simulink model "Regressao6_Comp"  (R2012b)
settings: Solver=FixedStepDiscrete  SolverMode=SingleTasking  StartTime=0.0  StopTime=buffer*limSim  FixedStep=ts  RelTol=1e-3
undefined symbols (not defined in the file): buffer, limSim, magnitude, ts
libraries: xbsIndex_r4 x52, dspstat3 x1, simulink x1, roblocks x1
settings Model: Creator=snata  LastModifiedBy=snata

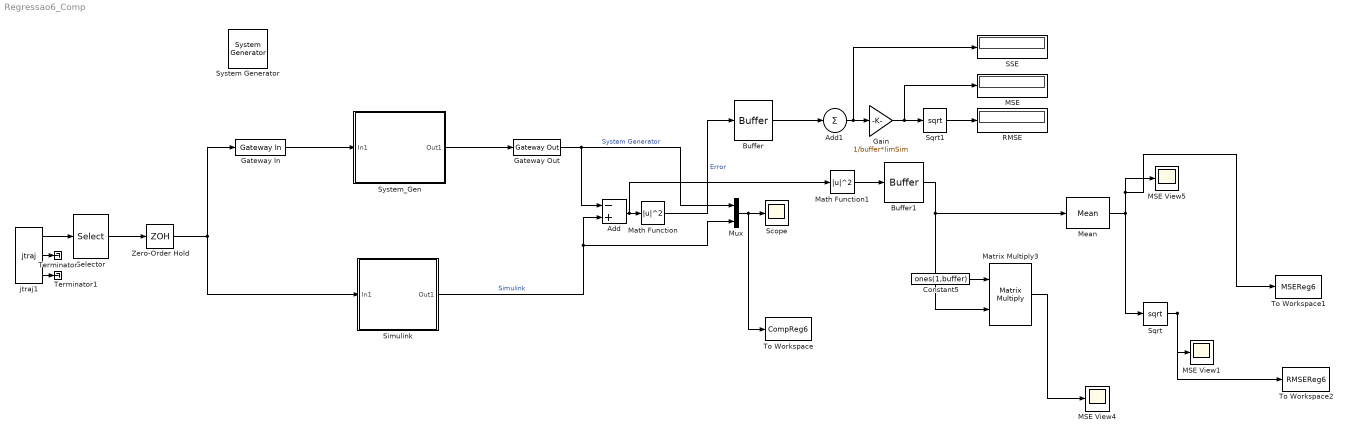
== system Regressao6_Comp ==
  " System Generator" : xbsIndex_r4/ System Generator  Tag=genX  xilinxfamily=virtex6  part=xc6vlx240t  speed=-1  package=ff1156  synthesis_tool=XST  clock_wrapper=Clock Enables  directory=./netlist  proj_type=Project Navigator  Synth_file=XST Defaults  Impl_file=ISE Defaults  testbench=off  simulink_period=ts  sysclk_period=10  dcm_input_clock_period=10  incr_netlist=off  trim_vbits=Everywhere in SubSystem  dbl_ovrd=According to Block Masks  core_generation=According to Block Masks  run_coregen=off  deprecated_control=off  eval_field=0  block_type=sysgen
  Add : Sum  Inputs=-+
  Add1 : Sum  Inputs=1
  Buffer : Buffer  N=buffer*limSim  TreatMby1Signals=One channel
  Buffer1 : Buffer  N=buffer  TreatMby1Signals=One channel
  Constant5 : Constant  Value=ones(1,buffer)  VectorParams1D=off
  Gain : Gain  Gain=1/buffer*limSim
  Gateway In : xbsIndex_r4/Gateway In  gui_display_data_type=Floating-point  arith_type=Floating-point  n_bits=16  bin_pt=14  preci_type=Single  exp_width=8  frac_width=24  quantization="Round  (unbiased: +/- Inf)"  overflow=Saturate  period=ts  dbl_ovrd=off  timing_constraint=None  locs_specified=off  LOCs={}  UseAsADC=off  ADCChannel='1'  inherit_from_input=off  hdl_port=on  block_type=gatewayin
  Gateway Out : xbsIndex_r4/Gateway Out  inherit_from_input=off  hdl_port=on  timing_constraint=None  locs_specified=off  LOCs={}  UseAsDAC=off  DACChannel='1'  block_type=gatewayout
  MSE : Display
  MSE View1 : Scope
      settings: TimeRange=1600  YMin=0.3388218390804599  YMax=0.5988218390804599  SaveName=ScopeData4  MaxDataPoints=5000000
  MSE View4 : Scope
      settings: TimeRange=1600  YMin=0.3388218390804599  YMax=0.5988218390804599  SaveName=ScopeData5  MaxDataPoints=5000000
  MSE View5 : Scope
      settings: ShowLegends=on  TimeRange=4000  YMin=0.3388218390804599  YMax=0.5988218390804599  SaveName=ScopeData6  MaxDataPoints=5000000
  Math Function1 : Math  Operator=magnitude^2  SaturateOnIntegerOverflow=on
  Math Function : Math  Operator=magnitude^2  SaturateOnIntegerOverflow=on
  Matrix Multiply3 : Product  Multiplication=Matrix(*)
  Mean : dspstat3/Mean  run=off  reset_popup=None  InputProcessing=Columns as channels (frame based)  directionMode=Each column  dimension=1  treatSBRowAsCol=on  roiEnable=off  roiType=Rectangles  roiPortion=Entire ROI  roiOutput=Individual statistics for each ROI  roiFlag=off  outputDataTypeStr=Inherit: Same as accumulator  outputLastDataTypeStr=Inherit: Same as accumulator  outputMin=[]  outputMax=[]  roundingMode=Floor  overflowMode=off
  Mux : Mux  Inputs=2
  RMSE : Display
  SSE : Display
  Scope : Scope
      settings: ShowLegends=on  TimeRange=40  YMin=0  YMax=200  MaxDataPoints=50000
  Selector : Selector  InputPortWidth=3  IndexOptions=Index vector (dialog)  Indices=[1]  OutputSizes=1
  Simulink : Subsystem
  Sqrt : Sqrt  SaturateOnIntegerOverflow=on
  Sqrt1 : Sqrt  SaturateOnIntegerOverflow=on
  System_Gen : Subsystem
  Terminator : Terminator
  Terminator1 : Terminator
  To Workspace : ToWorkspace  VariableName=CompReg6  SampleTime=-1
  To Workspace1 : ToWorkspace  VariableName=MSEReg6  SampleTime=-1
  To Workspace2 : ToWorkspace  VariableName=RMSEReg6  SampleTime=-1
  Zero-Order Hold : ZeroOrderHold  SampleTime=ts
  jtraj1 : roblocks/Trajectory/jtraj  q0=[0 -pi/2 pi]  qf=[pi/2 pi/4 pi/2]  tmax=buffer*limSim  ts=ts
  wires:
  Selector/1 -> Zero-Order Hold/1
  jtraj1/1 -> Selector/1
  Gateway In/1 -> System_Gen/1(In1)
  System_Gen/1(Out1) -> Gateway Out/1
  Gateway Out/1 -> Add/1, Mux/1  "System Generator"
  Simulink/1(Out1) -> Mux/2, Add/2  "Simulink"
  Zero-Order Hold/1 -> Gateway In/1, Simulink/1(In1)
  Math Function/1 -> Buffer/1  "Error"
  Gain/1 -> MSE/1, Sqrt1/1
  Buffer/1 -> Add1/1
  Add1/1 -> SSE/1, Gain/1
  Sqrt1/1 -> RMSE/1
  jtraj1/2 -> Terminator/1
  jtraj1/3 -> Terminator1/1
  Mux/1 -> To Workspace/1, Scope/1
  Add/1 -> Math Function1/1, Math Function/1
  Math Function1/1 -> Buffer1/1
  Buffer1/1 -> Mean/1, Matrix Multiply3/2
  Matrix Multiply3/1 -> MSE View4/1
  Constant5/1 -> Matrix Multiply3/1
  Mean/1 -> To Workspace1/1, MSE View5/1, Sqrt/1
  Sqrt/1 -> To Workspace2/1, MSE View1/1

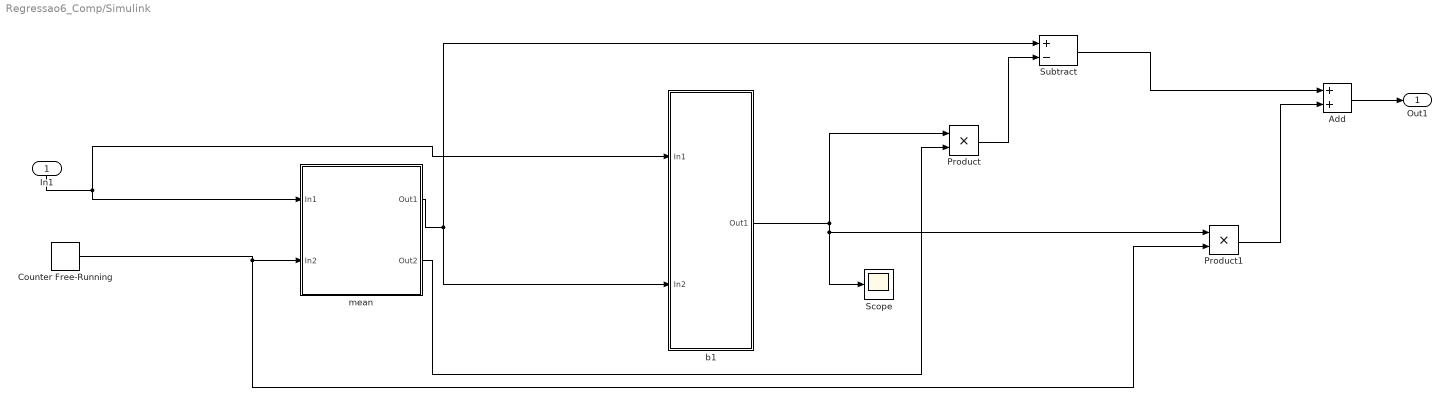
== system Regressao6_Comp/Simulink ==
  In1 : Inport
  Add : Sum
  Counter Free-Running : simulink/Sources/Counter Free-Running  NumBits=32  tsamp=ts
  Product : Product  RndMeth=Zero
  Product1 : Product  RndMeth=Zero
  Scope : Scope
      settings: ShowLegends=on  TimeRange=40  YMin=2.88  YMax=2.945  SaveName=ScopeData3  MaxDataPoints=50000
  Subtract : Sum  Inputs=+-
  b1 : Subsystem
  "mean " : Subsystem
  Out1 : Outport
  wires:
  Subtract/1 -> Add/1
  In1/1 -> "mean "/1(In1), b1/1(In1)
  Add/1 -> Out1/1
  "mean "/1(Out1) -> Subtract/1, b1/2(In2)
  b1/1(Out1) -> Scope/1, Product1/1, Product/1
  Counter Free-Running/1 -> "mean "/2(In2), Product1/2
  "mean "/2(Out2) -> Product/2
  Product/1 -> Subtract/2
  Product1/1 -> Add/2

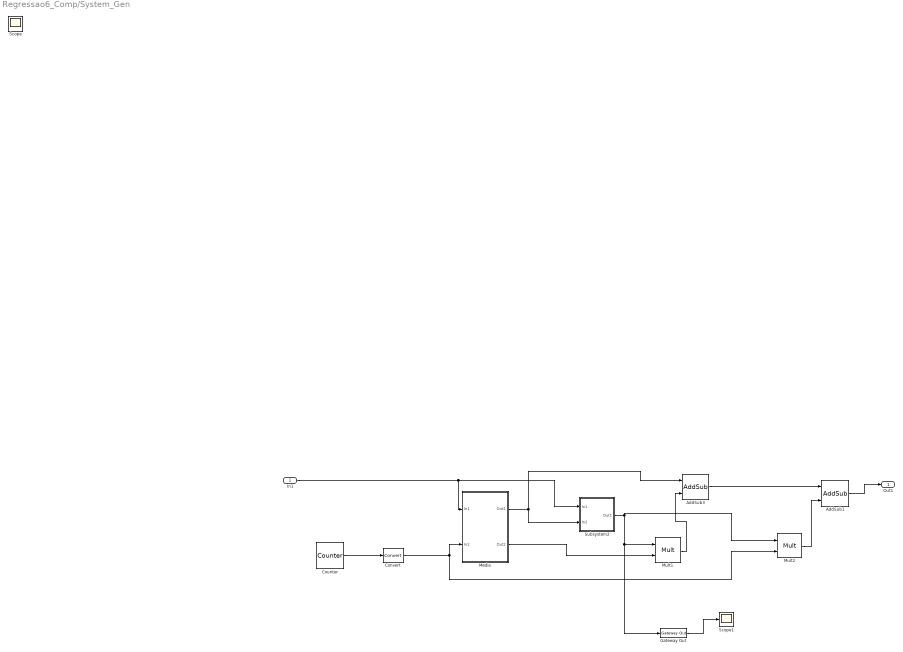
== system Regressao6_Comp/System_Gen ==
  In1 : Inport
  AddSub1 : xbsIndex_r4/AddSub  mode=Addition  use_carryin=off  use_carryout=off  en=off  latency=0  precision=Full  arith_type=Unsigned  n_bits=16  bin_pt=14  quantization=Truncate  overflow=Wrap  dbl_ovrd=off  use_behavioral_HDL=off  hw_selection=Fabric  pipelined=off  block_type=addsub
  AddSub3 : xbsIndex_r4/AddSub  mode=Subtraction  use_carryin=off  use_carryout=off  en=off  latency=0  precision=Full  arith_type=Unsigned  n_bits=16  bin_pt=14  quantization=Truncate  overflow=Wrap  dbl_ovrd=off  use_behavioral_HDL=off  hw_selection=Fabric  pipelined=off  block_type=addsub
  Convert : xbsIndex_r4/Convert  gui_display_data_type=Floating-point  arith_type=Floating-point  n_bits=16  bin_pt=14  float_type=Single  exp_bits=8  fraction_bits=24  quantization=Truncate  overflow=Wrap  en=off  latency=0  dbl_ovrd=off  pipeline=off  block_type=convert
  Counter : xbsIndex_r4/Counter  cnt_type=Free Running  cnt_to=Inf  operation=Up  start_count=0  cnt_by_val=1  arith_type="Signed  (2's comp)"  n_bits=32  bin_pt=0  load_pin=off  rst=off  en=off  explicit_period=on  period=ts  dbl_ovrd=off  use_behavioral_HDL=off  implementation=Fabric  block_type=counter
  Gateway Out : xbsIndex_r4/Gateway Out  inherit_from_input=off  hdl_port=on  timing_constraint=None  locs_specified=off  LOCs={}  UseAsDAC=off  DACChannel='1'  block_type=gatewayout
  "Media " : Subsystem
  Mult1 : xbsIndex_r4/Mult  precision=Full  arith_type="Signed  (2's comp)"  n_bits=16  bin_pt=14  quantization=Truncate  overflow=Wrap  en=off  latency=0  dbl_ovrd=off  use_behavioral_HDL=off  opt=Speed  use_embedded=on  optimum_pipeline=off  pipeline=on  use_rpm=on  placement_style=Triangular  block_type=mult
  Mult2 : xbsIndex_r4/Mult  precision=Full  arith_type="Signed  (2's comp)"  n_bits=16  bin_pt=14  quantization=Truncate  overflow=Wrap  en=off  latency=0  dbl_ovrd=off  use_behavioral_HDL=off  opt=Speed  use_embedded=on  optimum_pipeline=off  pipeline=on  use_rpm=on  placement_style=Triangular  block_type=mult
  Scope : Scope
      settings: ShowLegends=on  TimeRange=40  YMin=0  YMax=200  MaxDataPoints=50000
  Scope1 : Scope
      settings: ShowLegends=on  TimeRange=40  YMin=0  YMax=200  SaveName=ScopeData2  MaxDataPoints=50000
  Subsystem2 : Subsystem
  Out1 : Outport
  wires:
  AddSub1/1 -> Out1/1
  In1/1 -> Subsystem2/1(In1), "Media "/1(In1)
  "Media "/1(Out1) -> Subsystem2/2(In2), AddSub3/1
  Mult1/1 -> AddSub3/2
  AddSub3/1 -> AddSub1/1
  Mult2/1 -> AddSub1/2
  Subsystem2/1(Out1) -> Mult2/1, Gateway Out/1, Mult1/1
  "Media "/2(Out2) -> Mult1/2
  Counter/1 -> Convert/1
  Convert/1 -> "Media "/2(In2), Mult2/2
  Gateway Out/1 -> Scope1/1

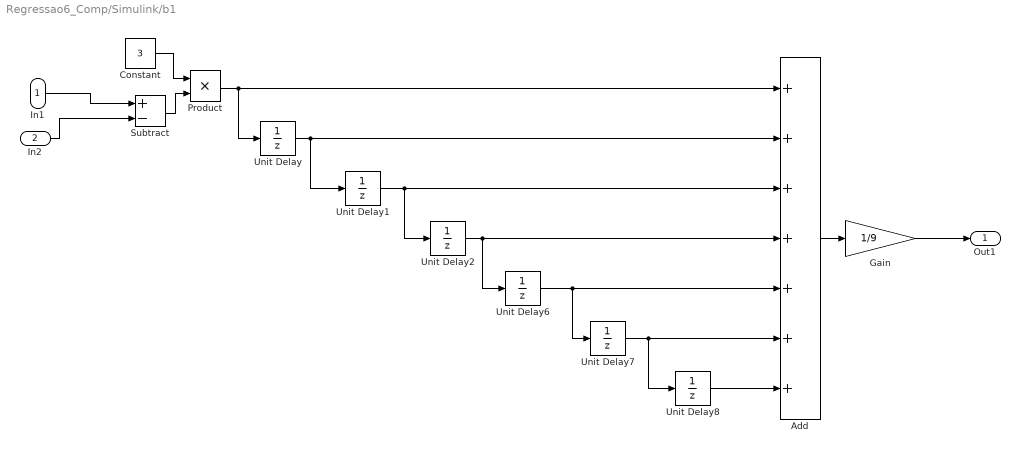
== system Regressao6_Comp/Simulink/b1 ==
  In1 : Inport
  In2 : Inport  Port=2
  Add : Sum  Inputs=+++++++
  Constant : Constant  Value=3
  Gain : Gain  Gain=1/9
  Product : Product
  Subtract : Sum  Inputs=+-
  Unit Delay{,1..2,6..8} (6 alike) : UnitDelay  SampleTime=-1
  Out1 : Outport
  wires:
  In1/1 -> Subtract/1
  Gain/1 -> Out1/1
  In2/1 -> Subtract/2
  Subtract/1 -> Product/2
  Add/1 -> Gain/1
  Constant/1 -> Product/1
  Unit Delay8/1 -> Add/7
  Unit Delay7/1 -> Unit Delay8/1, Add/6
  Unit Delay6/1 -> Unit Delay7/1, Add/5
  Unit Delay2/1 -> Unit Delay6/1, Add/4
  Unit Delay1/1 -> Unit Delay2/1, Add/3
  Unit Delay/1 -> Unit Delay1/1, Add/2
  Product/1 -> Unit Delay/1, Add/1

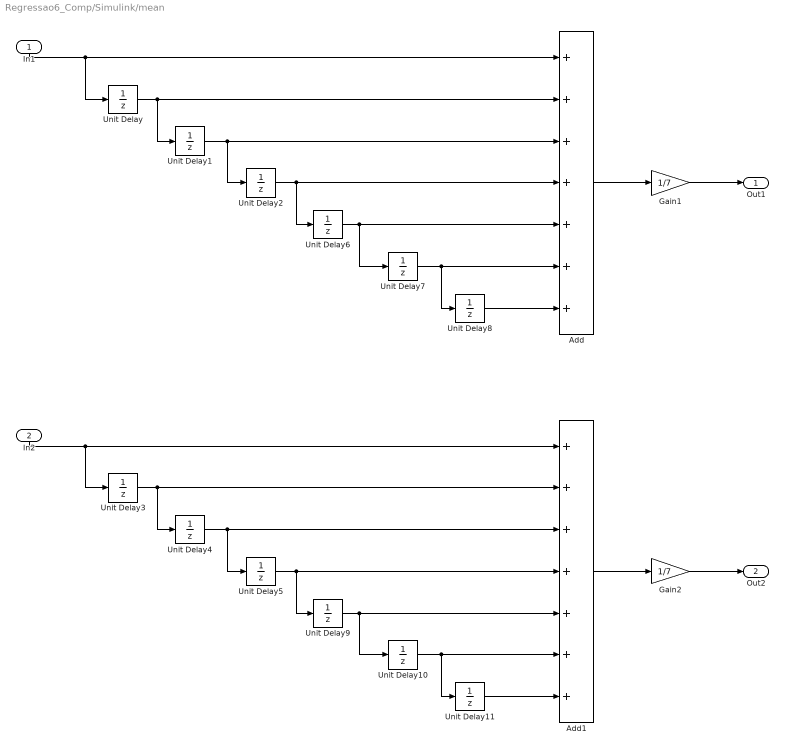
== system Regressao6_Comp/Simulink/mean  ==
  In1 : Inport
  In2 : Inport  Port=2
  Add : Sum  Inputs=+++++++
  Add1 : Sum  Inputs=+++++++
  Gain1 : Gain  Gain=1/7
  Gain2 : Gain  Gain=1/7
  Unit Delay{,1..11} (12 alike) : UnitDelay  SampleTime=-1
  Out1 : Outport
  Out2 : Outport  Port=2
  wires:
  Gain1/1 -> Out1/1
  Add/1 -> Gain1/1
  Unit Delay8/1 -> Add/7
  Unit Delay7/1 -> Unit Delay8/1, Add/6
  Unit Delay6/1 -> Unit Delay7/1, Add/5
  Unit Delay2/1 -> Unit Delay6/1, Add/4
  Unit Delay1/1 -> Unit Delay2/1, Add/3
  Unit Delay/1 -> Unit Delay1/1, Add/2
  In1/1 -> Unit Delay/1, Add/1
  Gain2/1 -> Out2/1
  Add1/1 -> Gain2/1
  Unit Delay11/1 -> Add1/7
  Unit Delay10/1 -> Add1/6, Unit Delay11/1
  Unit Delay9/1 -> Add1/5, Unit Delay10/1
  Unit Delay5/1 -> Add1/4, Unit Delay9/1
  Unit Delay4/1 -> Add1/3, Unit Delay5/1
  Unit Delay3/1 -> Add1/2, Unit Delay4/1
  In2/1 -> Add1/1, Unit Delay3/1

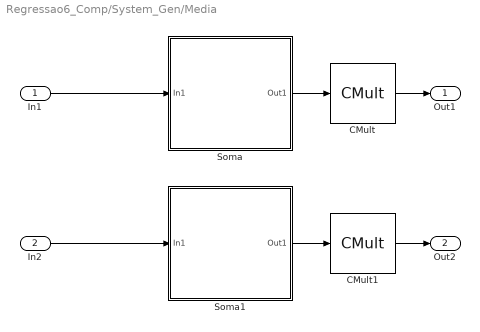
== system Regressao6_Comp/System_Gen/Media  ==
  In1 : Inport
  In2 : Inport  Port=2
  CMult : xbsIndex_r4/CMult  const=1/7  gui_display_data_type=Floating-point  const_n_bits=16  const_bin_pt=14  float_type=Single  exp_bits=8  fraction_bits=24  en=off  latency=0  precision=Full  arith_type="Signed  (2's comp)"  n_bits=16  bin_pt=14  quantization=Truncate  overflow=Wrap  dbl_ovrd=off  use_behavioral_HDL=off  mem_type=Distributed RAM  pipeline=off  block_type=cmult
  CMult1 : xbsIndex_r4/CMult  const=1/7  gui_display_data_type=Floating-point  const_n_bits=16  const_bin_pt=14  float_type=Single  exp_bits=8  fraction_bits=24  en=off  latency=0  precision=Full  arith_type="Signed  (2's comp)"  n_bits=16  bin_pt=14  quantization=Truncate  overflow=Wrap  dbl_ovrd=off  use_behavioral_HDL=off  mem_type=Distributed RAM  pipeline=off  block_type=cmult
  Soma : Subsystem
  Soma1 : Subsystem
  Out1 : Outport
  Out2 : Outport  Port=2
  wires:
  In1/1 -> Soma/1(In1)
  Soma/1(Out1) -> CMult/1
  CMult/1 -> Out1/1
  In2/1 -> Soma1/1(In1)
  Soma1/1(Out1) -> CMult1/1
  CMult1/1 -> Out2/1

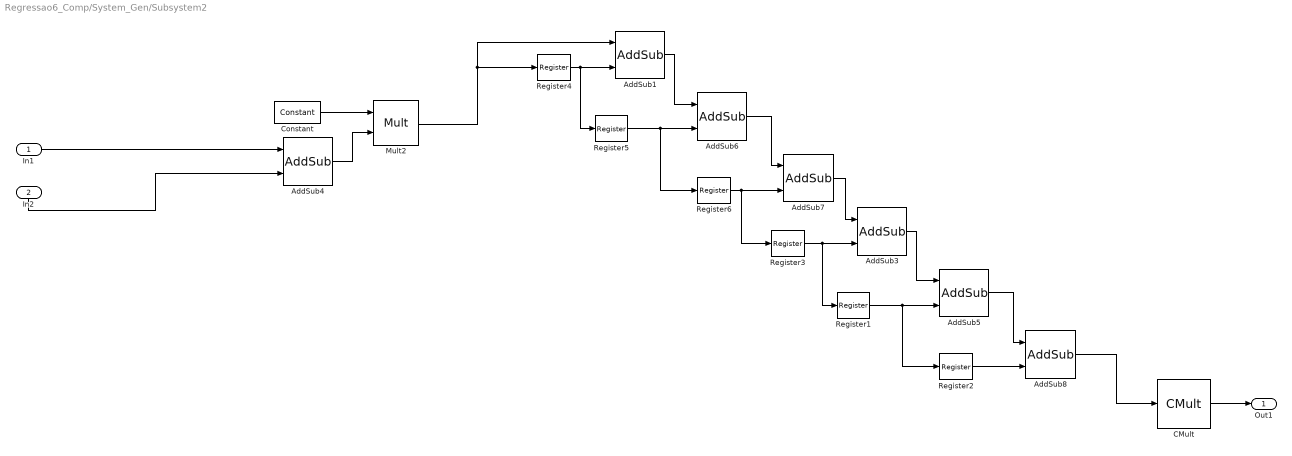
== system Regressao6_Comp/System_Gen/Subsystem2 ==
  In1 : Inport
  In2 : Inport  Port=2
  AddSub{1,3,5..8} (6 alike) : xbsIndex_r4/AddSub  mode=Addition  use_carryin=off  use_carryout=off  en=off  latency=0  precision=Full  arith_type=Unsigned  n_bits=16  bin_pt=14  quantization=Truncate  overflow=Wrap  dbl_ovrd=off  use_behavioral_HDL=off  hw_selection=Fabric  pipelined=off  block_type=addsub
  AddSub4 : xbsIndex_r4/AddSub  mode=Subtraction  use_carryin=off  use_carryout=off  en=off  latency=0  precision=Full  arith_type=Unsigned  n_bits=16  bin_pt=14  quantization=Truncate  overflow=Wrap  dbl_ovrd=off  use_behavioral_HDL=off  hw_selection=Fabric  pipelined=off  block_type=addsub
  CMult : xbsIndex_r4/CMult  const=1/9  gui_display_data_type=Floating-point  const_n_bits=16  const_bin_pt=14  float_type=Single  exp_bits=8  fraction_bits=24  en=off  latency=0  precision=Full  arith_type="Signed  (2's comp)"  n_bits=16  bin_pt=14  quantization=Truncate  overflow=Wrap  dbl_ovrd=off  use_behavioral_HDL=off  mem_type=Distributed RAM  pipeline=off  block_type=cmult
  Constant : xbsIndex_r4/Constant  const=3  gui_display_data_type=Floating-point  arith_type=Floating-point  n_bits=16  bin_pt=14  preci_type=Single  exp_width=8  frac_width=24  explicit_period=off  period=1  equ=P=C  opselect=C  inp2=PCIN>>17  opr=+  inp1=P  carry=CIN  dbl_ovrd=off  block_type=constant
  Mult2 : xbsIndex_r4/Mult  precision=Full  arith_type="Signed  (2's comp)"  n_bits=16  bin_pt=14  quantization=Truncate  overflow=Wrap  en=off  latency=0  dbl_ovrd=off  use_behavioral_HDL=off  opt=Speed  use_embedded=on  optimum_pipeline=off  pipeline=on  use_rpm=on  placement_style=Triangular  block_type=mult
  Register{1..6} (6 alike) : xbsIndex_r4/Register  init=0  rst=off  en=off  dbl_ovrd=off  block_type=register
  Out1 : Outport
  wires:
  Constant/1 -> Mult2/1
  AddSub7/1 -> AddSub3/1
  Register2/1 -> AddSub8/2
  Register1/1 -> AddSub5/2, Register2/1
  Register3/1 -> AddSub3/2, Register1/1
  AddSub3/1 -> AddSub5/1
  AddSub5/1 -> AddSub8/1
  Register6/1 -> AddSub7/2, Register3/1
  Register5/1 -> AddSub6/2, Register6/1
  Register4/1 -> AddSub1/2, Register5/1
  AddSub1/1 -> AddSub6/1
  AddSub6/1 -> AddSub7/1
  Mult2/1 -> Register4/1, AddSub1/1
  AddSub8/1 -> CMult/1
  In2/1 -> AddSub4/2
  In1/1 -> AddSub4/1
  AddSub4/1 -> Mult2/2
  CMult/1 -> Out1/1

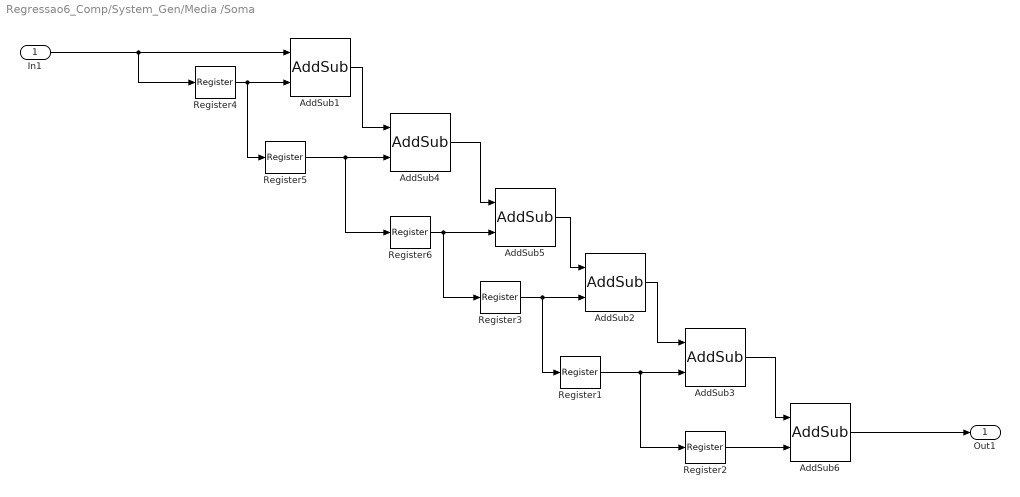
== system Regressao6_Comp/System_Gen/Media /Soma ==
  In1 : Inport
  AddSub{1..6} (6 alike) : xbsIndex_r4/AddSub  mode=Addition  use_carryin=off  use_carryout=off  en=off  latency=0  precision=Full  arith_type=Unsigned  n_bits=16  bin_pt=14  quantization=Truncate  overflow=Wrap  dbl_ovrd=off  use_behavioral_HDL=off  hw_selection=Fabric  pipelined=off  block_type=addsub
  Register{1..6} (6 alike) : xbsIndex_r4/Register  init=0  rst=off  en=off  dbl_ovrd=off  block_type=register
  Out1 : Outport
  wires:
  In1/1 -> Register4/1, AddSub1/1
  AddSub4/1 -> AddSub5/1
  AddSub1/1 -> AddSub4/1
  Register4/1 -> Register5/1, AddSub1/2
  Register5/1 -> Register6/1, AddSub4/2
  Register6/1 -> Register3/1, AddSub5/2
  AddSub3/1 -> AddSub6/1
  AddSub2/1 -> AddSub3/1
  Register3/1 -> Register1/1, AddSub2/2
  Register1/1 -> Register2/1, AddSub3/2
  Register2/1 -> AddSub6/2
  AddSub5/1 -> AddSub2/1
  AddSub6/1 -> Out1/1

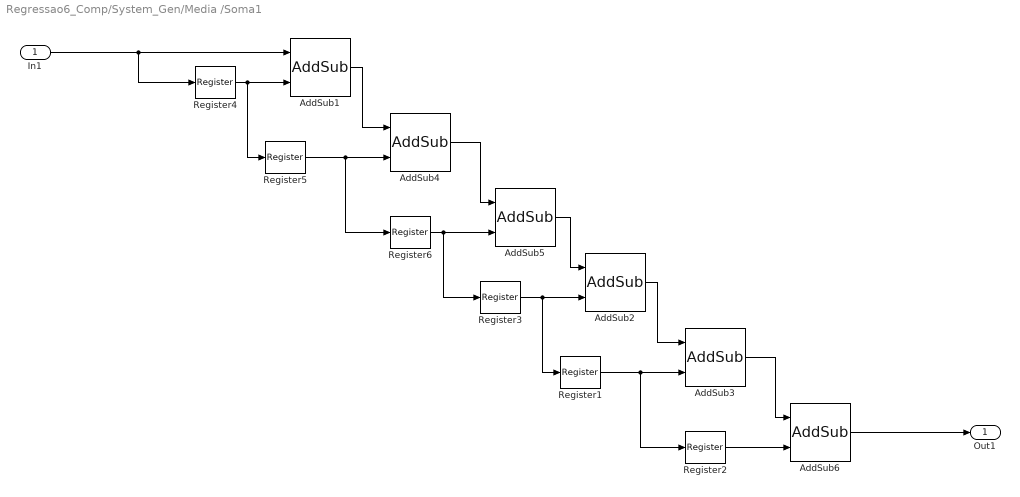
== system Regressao6_Comp/System_Gen/Media /Soma1 ==
  In1 : Inport
  AddSub{1..6} (6 alike) : xbsIndex_r4/AddSub  mode=Addition  use_carryin=off  use_carryout=off  en=off  latency=0  precision=Full  arith_type=Unsigned  n_bits=16  bin_pt=14  quantization=Truncate  overflow=Wrap  dbl_ovrd=off  use_behavioral_HDL=off  hw_selection=Fabric  pipelined=off  block_type=addsub
  Register{1..6} (6 alike) : xbsIndex_r4/Register  init=0  rst=off  en=off  dbl_ovrd=off  block_type=register
  Out1 : Outport
  wires:
  AddSub6/1 -> Out1/1
  AddSub5/1 -> AddSub2/1
  Register2/1 -> AddSub6/2
  Register1/1 -> AddSub3/2, Register2/1
  Register3/1 -> AddSub2/2, Register1/1
  AddSub2/1 -> AddSub3/1
  AddSub3/1 -> AddSub6/1
  Register6/1 -> AddSub5/2, Register3/1
  Register5/1 -> AddSub4/2, Register6/1
  Register4/1 -> AddSub1/2, Register5/1
  AddSub1/1 -> AddSub4/1
  AddSub4/1 -> AddSub5/1
  In1/1 -> AddSub1/1, Register4/1
